simulink model "Experiment_cs"  (Simulink 8.4)
settings: Solver=ode5  SolverMode=SingleTasking  StartTime=0.0  StopTime=inf  FixedStep=1/100  RelTol=1e-3
PreLoadFcn:
  | mbxruntime.callbacks.PreLoadFcn(bdroot);
PostLoadFcn:
  | mbxruntime.callbacks.PostLoadFcn(bdroot);
InitFcn:
  | mbxruntime.callbacks.InitFcn(bdroot);
StartFcn:
  | mbxruntime.callbacks.StartFcn(bdroot);
StopFcn:
  | mbxruntime.callbacks.StopFcn(bdroot);
undefined symbols (not defined in the file or in its folder): dfreq, gray, InitImageOutputDir, Rec, SDTV, strel
libraries: simulink x79, visiontextngfix x30, simulink_extras x23, PreScanSimulinkLibrary x20, visionconversions x6, visionsinks x4, PreScanUsefulBlocks x3, visionstatistics x2, visionmorphops x2, visionanalysis x2, simulink_need_slupdate x2
(part 10 of 11)

== system Experiment_cs/Audi_A8_1/ENABLED/Dynamics_Simple/Chassis/Bicycle_model_[XYZ]/X_Motion/BrakeSystem ==
  vx_[ms-1] : Inport
  BrakePressure_[bar] : Inport  Port=2
  Gain : Gain  Gain=1/p.Rw
  Saturation : Saturate  UpperLimit=p.PBrakeMax  LowerLimit=0
  Saturation1 : Saturate  UpperLimit=5/15  LowerLimit=-5/15
  Sign : Signum
  "[ms-1] 2 [rads-1]" : Gain  Gain=1/p.Rw  SaturateOnIntegerOverflow=on  OutDataTypeStr=Inherit: Same as input  ParamDataTypeStr=Inherit: Same as input
  braking Q factor : Gain  Gain=p.Qfac  SaturateOnIntegerOverflow=on  OutDataTypeStr=Inherit: Same as input  ParamDataTypeStr=Inherit: Same as input
  signed load1 : Product  SaturateOnIntegerOverflow=on  InputSameDT=on  OutDataTypeStr=Inherit: Same as first input
  BrakeForce : Outport
  BrakeTorqueAbs : Outport  Port=2
  wires:
  braking Q factor/1 -> BrakeTorqueAbs/1, Gain/1
  BrakePressure_[bar]/1 -> Saturation/1
  Saturation/1 -> braking Q factor/1
  vx_[ms-1]/1 -> "[ms-1] 2 [rads-1]"/1
  Saturation1/1 -> Sign/1
  "[ms-1] 2 [rads-1]"/1 -> Saturation1/1
  Sign/1 -> signed load1/2  "sign"
  signed load1/1 -> BrakeForce/1
  Gain/1 -> signed load1/1

== system Experiment_cs/Audi_A8_1/ENABLED/Dynamics_Simple/Chassis/Bicycle_model_[XYZ]/X_Motion/Configurable Subsystem ==
  In1 : Inport
  In2 : Inport  Port=2
  In3 : Inport  Port=3
  Integrator : Integrator  ExternalReset=level  InitialConditionSource=external
  Out1 : Outport
  wires:
  In1/1 -> Integrator/1
  In2/1 -> Integrator/2
  In3/1 -> Integrator/3
  Integrator/1 -> Out1/1

== system Experiment_cs/Audi_A8_1/ENABLED/Dynamics_Simple/Chassis/Bicycle_model_[XYZ]/X_Motion/Configurable Subsystem1 ==
  In1 : Inport
  Torsional damping : TransferFcn  Denominator=[0.1 1]
  Out1 : Outport
  wires:
  In1/1 -> Torsional damping/1
  Torsional damping/1 -> Out1/1

== system Experiment_cs/Audi_A8_1/ENABLED/Dynamics_Simple/Chassis/Bicycle_model_[XYZ]/X_Motion/Max RPM and zero- velocity detection ==
  note: Set to zero after infinite small time-step
  note: Zero velocity detection
  ax : Inport
  Drive Torque : Inport  Port=2
  Brake Torque : Inport  Port=3
  v0 : Inport  Port=4
  vx : Inport  Port=5
  Abs : Abs
  Abs1 : Abs
  Compare To Zero : simulink/Logic and Bit Operations/Compare To Zero  relop=<=  OutDataTypeStr=boolean  ZeroCross=off
  Compare To Zero1 : simulink/Logic and Bit Operations/Compare To Zero  relop=>=  OutDataTypeStr=boolean  ZeroCross=off
  Compare To Zero2 : simulink/Logic and Bit Operations/Compare To Zero  relop=>=  OutDataTypeStr=boolean  ZeroCross=off
  Compare To Zero3 : simulink/Logic and Bit Operations/Compare To Zero  relop=<=  OutDataTypeStr=boolean  ZeroCross=off
  Configurable Subsystem : Subsystem  BlockChoice=Step  mask{ComputationMode=ComputationMode}
      mask prompts: ComputationMode "Compuation mode:"
      mask init:
      | SetComputationMode(gcb,ComputationMode);
      settings: AttributesFormatString=%<BlockChoice>  OpenFcn=BringToFront(gcb);  MemberBlocks=Discrete Step,Step
      settings: TemplateBlock=|
      | PreScanSimulinkLibrary/Configurable Subsystems/Step Function/Configurable
      | Subsystem
  Constant : Constant
  Constant1 : Constant
  Logical Operator : Logic  AllPortsSameDT=off  OutDataTypeStr=boolean
  Logical Operator1 : Logic  AllPortsSameDT=off  OutDataTypeStr=boolean
  Logical Operator2 : Logic  Operator=NOT  AllPortsSameDT=off  OutDataTypeStr=boolean
  Logical Operator3 : Logic  AllPortsSameDT=off  OutDataTypeStr=boolean
  Logical Operator4 : Logic  Operator=OR  AllPortsSameDT=off  OutDataTypeStr=boolean
  Memory : Memory
  Memory1 : Memory
  Memory2 : Memory
  Product : Product  RndMeth=Zero
  Relational Operator : RelationalOperator  Operator=<  OutDataTypeStr=boolean
  SR-Memory : Subsystem
  Sum : Sum  Inputs=|-+
  Switch : Switch  Criteria=u2 ~= 0  Threshold=0.5
  ax is 0 : Constant  Value=0
  ax_out : Outport
  vx_reset : Outport  Port=2
  x0 : Outport  Port=3
  wires:
  Logical Operator4/1 -> Logical Operator1/1
  vx/1 -> Compare To Zero/1, Compare To Zero2/1, Memory2/1, Memory/1  "vx"
  Memory2/1 -> Compare To Zero3/1
  Compare To Zero2/1 -> Logical Operator3/1
  Compare To Zero3/1 -> Logical Operator3/2
  Logical Operator3/1 -> Logical Operator4/2  "zero-crossing backward"
  Memory/1 -> Compare To Zero1/1
  Compare To Zero/1 -> Logical Operator/1
  Compare To Zero1/1 -> Logical Operator/2
  Logical Operator/1 -> Logical Operator4/1  "zero-crossing forward"
  Abs/1 -> Relational Operator/1
  Abs1/1 -> Relational Operator/2
  Drive Torque/1 -> Abs/1
  Brake Torque/1 -> Abs1/1
  Relational Operator/1 -> Logical Operator1/2, Logical Operator2/1
  Logical Operator1/1 -> SR-Memory/2(Set)
  Constant/1 -> SR-Memory/1(Signal)
  Logical Operator2/1 -> SR-Memory/3(Reset)
  SR-Memory/1(Out) -> Sum/1, Memory1/1
  Switch/1 -> ax_out/1
  Sum/1 -> Switch/2
  ax is 0/1 -> Switch/3
  Constant1/1 -> Sum/2
  v0/1 -> Product/1
  Product/1 -> x0/1
  Configurable Subsystem/1(Out1) -> Product/2
  ax/1 -> Switch/1  "ax"
  Memory1/1 -> vx_reset/1  "vx"

== system Experiment_cs/Audi_A8_1/ENABLED/Dynamics_Simple/Chassis/Bicycle_model_[XYZ]/Y & Yaw_Motion/Configurable Subsystem ==
  In1 : Inport
  In2 : Inport  Port=2
  Integrator : Integrator  ExternalReset=level
  Out1 : Outport
  wires:
  In1/1 -> Integrator/1
  In2/1 -> Integrator/2
  Integrator/1 -> Out1/1

== system Experiment_cs/Audi_A8_1/ENABLED/Dynamics_Simple/Chassis/Bicycle_model_[XYZ]/Y & Yaw_Motion/Configurable Subsystem1 ==
  In1 : Inport
  Integrator : Integrator
  Out1 : Outport
  wires:
  In1/1 -> Integrator/1
  Integrator/1 -> Out1/1

== system Experiment_cs/Audi_A8_1/ENABLED/Dynamics_Simple/Chassis/Bicycle_model_[XYZ]/Y & Yaw_Motion/Configurable Subsystem2 ==
  In1 : Inport
  In2 : Inport  Port=2
  Integrator : Integrator  ExternalReset=level
  Out1 : Outport
  wires:
  In1/1 -> Integrator/1
  In2/1 -> Integrator/2
  Integrator/1 -> Out1/1

== system Experiment_cs/Audi_A8_1/ENABLED/Dynamics_Simple/Chassis/Bicycle_model_[XYZ]/Z, Pitch_Motion & Roll_Motion/Configurable Subsystem ==
  In1 : Inport
  Integrator : Integrator  LimitOutput=on  UpperSaturationLimit=5*pi/180  LowerSaturationLimit=-5*pi/180
  Out1 : Outport
  wires:
  In1/1 -> Integrator/1
  Integrator/1 -> Out1/1

== system Experiment_cs/Audi_A8_1/ENABLED/Dynamics_Simple/Chassis/Bicycle_model_[XYZ]/Z, Pitch_Motion & Roll_Motion/Configurable Subsystem1 ==
  In1 : Inport
  Integrator : Integrator
  Out1 : Outport
  wires:
  In1/1 -> Integrator/1
  Integrator/1 -> Out1/1

== system Experiment_cs/Audi_A8_1/ENABLED/Dynamics_Simple/Chassis/Bicycle_model_[XYZ]/Z, Pitch_Motion & Roll_Motion/Configurable Subsystem2 ==
  In1 : Inport
  Integrator : Integrator
  Out1 : Outport
  wires:
  In1/1 -> Integrator/1
  Integrator/1 -> Out1/1

== system Experiment_cs/Audi_A8_1/ENABLED/Dynamics_Simple/Chassis/Bicycle_model_[XYZ]/Z, Pitch_Motion & Roll_Motion/Configurable Subsystem3 ==
  In1 : Inport
  Integrator : Integrator
  Out1 : Outport
  wires:
  In1/1 -> Integrator/1
  Integrator/1 -> Out1/1

== system Experiment_cs/Audi_A8_1/ENABLED/Dynamics_Simple/Chassis/Bicycle_model_[XYZ]/Z, Pitch_Motion & Roll_Motion/Configurable Subsystem4 ==
  In1 : Inport
  Integrator : Integrator
  Out1 : Outport
  wires:
  In1/1 -> Integrator/1
  Integrator/1 -> Out1/1

== system Experiment_cs/Audi_A8_1/ENABLED/Dynamics_Simple/Chassis/Bicycle_model_[XYZ]/Z, Pitch_Motion & Roll_Motion/Configurable Subsystem5 ==
  In1 : Inport
  Integrator : Integrator
  Out1 : Outport
  wires:
  In1/1 -> Integrator/1
  Integrator/1 -> Out1/1

== system Experiment_cs/Audi_A8_1/ENABLED/Dynamics_Simple/Chassis/Bicycle_model_[XYZ]/Z, Pitch_Motion & Roll_Motion/Configurable Subsystem9 ==
  In1 : Inport
  Derivative : Derivative
  Out1 : Outport
  wires:
  In1/1 -> Derivative/1
  Derivative/1 -> Out1/1

== system Experiment_cs/Audi_A8_1/ENABLED/Dynamics_Simple/Chassis/FrontTyre/AlphaFront/Enabled Subsystem ==
  In : Inport
  Enable : EnablePort  PropagateVarSize=During execution
  AlphaFront : Fcn  Expr=-atan( (u(2)+u(3)*p.a)/u(1) )
  Alpha : Outport  OutputWhenDisabled=reset  InitialOutput=[0]
  wires:
  AlphaFront/1 -> Alpha/1
  In/1 -> AlphaFront/1

== system Experiment_cs/Audi_A8_1/ENABLED/Dynamics_Simple/Chassis/RearTyre/AlphaRear/Enabled Subsystem ==
  In : Inport
  Enable : EnablePort  PropagateVarSize=During execution
  AlphaRear : Fcn  Expr=-atan( (u(2)-u(3)*p.b)/u(1) )
  Alpha : Outport  OutputWhenDisabled=reset  InitialOutput=[0]
  wires:
  AlphaRear/1 -> Alpha/1
  In/1 -> AlphaRear/1

== system Experiment_cs/Audi_A8_1/ENABLED/Trajectories/Traj2State1/Traj2State2/Traj2MuxState_Ext/demux ==
  traj : Inport
  Demux : Demux  Outputs=18
  x : Outport
  y : Outport  Port=2
  z : Outport  Port=3
  velx : Outport  Port=4
  vely : Outport  Port=5
  velz : Outport  Port=6
  R : Outport  Port=7
  P : Outport  Port=8
  Y : Outport  Port=9
  velR : Outport  Port=10
  velP : Outport  Port=11
  velY : Outport  Port=12
  accx : Outport  Port=13
  accy : Outport  Port=14
  accz : Outport  Port=15
  accR : Outport  Port=16
  accP : Outport  Port=17
  accY : Outport  Port=18
  wires:
  Demux/18 -> accY/1
  Demux/17 -> accP/1
  Demux/16 -> accR/1
  Demux/15 -> accz/1
  Demux/14 -> accy/1
  Demux/13 -> accx/1
  Demux/12 -> velY/1
  Demux/11 -> velP/1
  Demux/10 -> velR/1
  Demux/9 -> velz/1
  Demux/8 -> vely/1
  Demux/7 -> velx/1
  Demux/6 -> Y/1
  Demux/5 -> P/1
  traj/1 -> Demux/1
  Demux/4 -> R/1
  Demux/3 -> z/1
  Demux/2 -> y/1
  Demux/1 -> x/1

== system Experiment_cs/BMW_Z3_1/ENABLED/Dynamics_Simple/Chassis/Bicycle_model_[XYZ]/X_Motion/Air&RoadResistance ==
  vx_[ms-1] : Inport
  Gain : Gain  Gain=1/p.Rw
  Road & Aerodyn Resistances : Fcn  Expr=p.Rroad + p.Rair*u^2
  Saturation1 : Saturate  UpperLimit=5/15  LowerLimit=-5/15
  Sign : Signum
  "[ms-1] 2 [rads-1]" : Gain  Gain=1/p.Rw  SaturateOnIntegerOverflow=on  OutDataTypeStr=Inherit: Same as input  ParamDataTypeStr=Inherit: Same as input
  signed load1 : Product  SaturateOnIntegerOverflow=on  InputSameDT=on  OutDataTypeStr=Inherit: Same as first input
  Resistance_Force : Outport
  wires:
  signed load1/1 -> Resistance_Force/1  "F_[N]"
  vx_[ms-1]/1 -> Road & Aerodyn Resistances/1, "[ms-1] 2 [rads-1]"/1
  Saturation1/1 -> Sign/1
  "[ms-1] 2 [rads-1]"/1 -> Saturation1/1
  Road & Aerodyn Resistances/1 -> Gain/1  "ResistanceTorque_[Nm]"
  Sign/1 -> signed load1/2  "sign"
  Gain/1 -> signed load1/1  "Resistance Force_[N]"

== system Experiment_cs/BMW_Z3_1/ENABLED/Dynamics_Simple/Chassis/Bicycle_model_[XYZ]/X_Motion/BrakeSystem ==
  vx_[ms-1] : Inport
  BrakePressure_[bar] : Inport  Port=2
  Gain : Gain  Gain=1/p.Rw
  Saturation : Saturate  UpperLimit=p.PBrakeMax  LowerLimit=0
  Saturation1 : Saturate  UpperLimit=5/15  LowerLimit=-5/15
  Sign : Signum
  "[ms-1] 2 [rads-1]" : Gain  Gain=1/p.Rw  SaturateOnIntegerOverflow=on  OutDataTypeStr=Inherit: Same as input  ParamDataTypeStr=Inherit: Same as input
  braking Q factor : Gain  Gain=p.Qfac  SaturateOnIntegerOverflow=on  OutDataTypeStr=Inherit: Same as input  ParamDataTypeStr=Inherit: Same as input
  signed load1 : Product  SaturateOnIntegerOverflow=on  InputSameDT=on  OutDataTypeStr=Inherit: Same as first input
  BrakeForce : Outport
  BrakeTorqueAbs : Outport  Port=2
  wires:
  braking Q factor/1 -> BrakeTorqueAbs/1, Gain/1
  BrakePressure_[bar]/1 -> Saturation/1
  Saturation/1 -> braking Q factor/1
  vx_[ms-1]/1 -> "[ms-1] 2 [rads-1]"/1
  Saturation1/1 -> Sign/1
  "[ms-1] 2 [rads-1]"/1 -> Saturation1/1
  Sign/1 -> signed load1/2  "sign"
  signed load1/1 -> BrakeForce/1
  Gain/1 -> signed load1/1

== system Experiment_cs/BMW_Z3_1/ENABLED/Dynamics_Simple/Chassis/Bicycle_model_[XYZ]/X_Motion/Configurable Subsystem ==
  In1 : Inport
  In2 : Inport  Port=2
  In3 : Inport  Port=3
  Integrator : Integrator  ExternalReset=level  InitialConditionSource=external
  Out1 : Outport
  wires:
  In1/1 -> Integrator/1
  In2/1 -> Integrator/2
  In3/1 -> Integrator/3
  Integrator/1 -> Out1/1

== system Experiment_cs/BMW_Z3_1/ENABLED/Dynamics_Simple/Chassis/Bicycle_model_[XYZ]/X_Motion/Configurable Subsystem1 ==
  In1 : Inport
  Torsional damping : TransferFcn  Denominator=[0.1 1]
  Out1 : Outport
  wires:
  In1/1 -> Torsional damping/1
  Torsional damping/1 -> Out1/1

== system Experiment_cs/BMW_Z3_1/ENABLED/Dynamics_Simple/Chassis/Bicycle_model_[XYZ]/X_Motion/Max RPM and zero- velocity detection ==
  note: Set to zero after infinite small time-step
  note: Zero velocity detection
  ax : Inport
  Drive Torque : Inport  Port=2
  Brake Torque : Inport  Port=3
  v0 : Inport  Port=4
  vx : Inport  Port=5
  Abs : Abs
  Abs1 : Abs
  Compare To Zero : simulink/Logic and Bit Operations/Compare To Zero  relop=<=  OutDataTypeStr=boolean  ZeroCross=off
  Compare To Zero1 : simulink/Logic and Bit Operations/Compare To Zero  relop=>=  OutDataTypeStr=boolean  ZeroCross=off
  Compare To Zero2 : simulink/Logic and Bit Operations/Compare To Zero  relop=>=  OutDataTypeStr=boolean  ZeroCross=off
  Compare To Zero3 : simulink/Logic and Bit Operations/Compare To Zero  relop=<=  OutDataTypeStr=boolean  ZeroCross=off
  Configurable Subsystem : Subsystem  BlockChoice=Step  mask{ComputationMode=ComputationMode}
      mask prompts: ComputationMode "Compuation mode:"
      mask init:
      | SetComputationMode(gcb,ComputationMode);
      settings: AttributesFormatString=%<BlockChoice>  OpenFcn=BringToFront(gcb);  MemberBlocks=Discrete Step,Step
      settings: TemplateBlock=|
      | PreScanSimulinkLibrary/Configurable Subsystems/Step Function/Configurable
      | Subsystem
  Constant : Constant
  Constant1 : Constant
  Logical Operator : Logic  AllPortsSameDT=off  OutDataTypeStr=boolean
  Logical Operator1 : Logic  AllPortsSameDT=off  OutDataTypeStr=boolean
  Logical Operator2 : Logic  Operator=NOT  AllPortsSameDT=off  OutDataTypeStr=boolean
  Logical Operator3 : Logic  AllPortsSameDT=off  OutDataTypeStr=boolean
  Logical Operator4 : Logic  Operator=OR  AllPortsSameDT=off  OutDataTypeStr=boolean
  Memory : Memory
  Memory1 : Memory
  Memory2 : Memory
  Product : Product  RndMeth=Zero
  Relational Operator : RelationalOperator  Operator=<  OutDataTypeStr=boolean
  SR-Memory : Subsystem
  Sum : Sum  Inputs=|-+
  Switch : Switch  Criteria=u2 ~= 0  Threshold=0.5
  ax is 0 : Constant  Value=0
  ax_out : Outport
  vx_reset : Outport  Port=2
  x0 : Outport  Port=3
  wires:
  Logical Operator4/1 -> Logical Operator1/1
  vx/1 -> Compare To Zero/1, Compare To Zero2/1, Memory2/1, Memory/1  "vx"
  Memory2/1 -> Compare To Zero3/1
  Compare To Zero2/1 -> Logical Operator3/1
  Compare To Zero3/1 -> Logical Operator3/2
  Logical Operator3/1 -> Logical Operator4/2  "zero-crossing backward"
  Memory/1 -> Compare To Zero1/1
  Compare To Zero/1 -> Logical Operator/1
  Compare To Zero1/1 -> Logical Operator/2
  Logical Operator/1 -> Logical Operator4/1  "zero-crossing forward"
  Abs/1 -> Relational Operator/1
  Abs1/1 -> Relational Operator/2
  Drive Torque/1 -> Abs/1
  Brake Torque/1 -> Abs1/1
  Relational Operator/1 -> Logical Operator1/2, Logical Operator2/1
  Logical Operator1/1 -> SR-Memory/2(Set)
  Constant/1 -> SR-Memory/1(Signal)
  Logical Operator2/1 -> SR-Memory/3(Reset)
  SR-Memory/1(Out) -> Sum/1, Memory1/1
  Switch/1 -> ax_out/1
  Sum/1 -> Switch/2
  ax is 0/1 -> Switch/3
  Constant1/1 -> Sum/2
  v0/1 -> Product/1
  Product/1 -> x0/1
  Configurable Subsystem/1(Out1) -> Product/2
  ax/1 -> Switch/1  "ax"
  Memory1/1 -> vx_reset/1  "vx"

== system Experiment_cs/BMW_Z3_1/ENABLED/Dynamics_Simple/Chassis/Bicycle_model_[XYZ]/Y & Yaw_Motion/Configurable Subsystem ==
  In1 : Inport
  In2 : Inport  Port=2
  Integrator : Integrator  ExternalReset=level
  Out1 : Outport
  wires:
  In1/1 -> Integrator/1
  In2/1 -> Integrator/2
  Integrator/1 -> Out1/1

== system Experiment_cs/BMW_Z3_1/ENABLED/Dynamics_Simple/Chassis/Bicycle_model_[XYZ]/Y & Yaw_Motion/Configurable Subsystem1 ==
  In1 : Inport
  Integrator : Integrator
  Out1 : Outport
  wires:
  In1/1 -> Integrator/1
  Integrator/1 -> Out1/1

== system Experiment_cs/BMW_Z3_1/ENABLED/Dynamics_Simple/Chassis/Bicycle_model_[XYZ]/Y & Yaw_Motion/Configurable Subsystem2 ==
  In1 : Inport
  In2 : Inport  Port=2
  Integrator : Integrator  ExternalReset=level
  Out1 : Outport
  wires:
  In1/1 -> Integrator/1
  In2/1 -> Integrator/2
  Integrator/1 -> Out1/1

== system Experiment_cs/BMW_Z3_1/ENABLED/Dynamics_Simple/Chassis/Bicycle_model_[XYZ]/Z, Pitch_Motion & Roll_Motion/Configurable Subsystem ==
  In1 : Inport
  Integrator : Integrator  LimitOutput=on  UpperSaturationLimit=5*pi/180  LowerSaturationLimit=-5*pi/180
  Out1 : Outport
  wires:
  In1/1 -> Integrator/1
  Integrator/1 -> Out1/1

== system Experiment_cs/BMW_Z3_1/ENABLED/Dynamics_Simple/Chassis/Bicycle_model_[XYZ]/Z, Pitch_Motion & Roll_Motion/Configurable Subsystem1 ==
  In1 : Inport
  Integrator : Integrator
  Out1 : Outport
  wires:
  In1/1 -> Integrator/1
  Integrator/1 -> Out1/1

== system Experiment_cs/BMW_Z3_1/ENABLED/Dynamics_Simple/Chassis/Bicycle_model_[XYZ]/Z, Pitch_Motion & Roll_Motion/Configurable Subsystem2 ==
  In1 : Inport
  Integrator : Integrator
  Out1 : Outport
  wires:
  In1/1 -> Integrator/1
  Integrator/1 -> Out1/1

== system Experiment_cs/BMW_Z3_1/ENABLED/Dynamics_Simple/Chassis/Bicycle_model_[XYZ]/Z, Pitch_Motion & Roll_Motion/Configurable Subsystem3 ==
  In1 : Inport
  Integrator : Integrator
  Out1 : Outport
  wires:
  In1/1 -> Integrator/1
  Integrator/1 -> Out1/1

== system Experiment_cs/BMW_Z3_1/ENABLED/Dynamics_Simple/Chassis/Bicycle_model_[XYZ]/Z, Pitch_Motion & Roll_Motion/Configurable Subsystem4 ==
  In1 : Inport
  Integrator : Integrator
  Out1 : Outport
  wires:
  In1/1 -> Integrator/1
  Integrator/1 -> Out1/1

== system Experiment_cs/BMW_Z3_1/ENABLED/Dynamics_Simple/Chassis/Bicycle_model_[XYZ]/Z, Pitch_Motion & Roll_Motion/Configurable Subsystem5 ==
  In1 : Inport
  Integrator : Integrator
  Out1 : Outport
  wires:
  In1/1 -> Integrator/1
  Integrator/1 -> Out1/1

== system Experiment_cs/BMW_Z3_1/ENABLED/Dynamics_Simple/Chassis/Bicycle_model_[XYZ]/Z, Pitch_Motion & Roll_Motion/Configurable Subsystem9 ==
  In1 : Inport
  Derivative : Derivative
  Out1 : Outport
  wires:
  In1/1 -> Derivative/1
  Derivative/1 -> Out1/1

== system Experiment_cs/BMW_Z3_1/ENABLED/Dynamics_Simple/Chassis/FrontTyre/AlphaFront/Enabled Subsystem ==
  In : Inport
  Enable : EnablePort  PropagateVarSize=During execution
  AlphaFront : Fcn  Expr=-atan( (u(2)+u(3)*p.a)/u(1) )
  Alpha : Outport  OutputWhenDisabled=reset  InitialOutput=[0]
  wires:
  AlphaFront/1 -> Alpha/1
  In/1 -> AlphaFront/1

== system Experiment_cs/BMW_Z3_1/ENABLED/Dynamics_Simple/Chassis/RearTyre/AlphaRear/Enabled Subsystem ==
  In : Inport
  Enable : EnablePort  PropagateVarSize=During execution
  AlphaRear : Fcn  Expr=-atan( (u(2)-u(3)*p.b)/u(1) )
  Alpha : Outport  OutputWhenDisabled=reset  InitialOutput=[0]
  wires:
  AlphaRear/1 -> Alpha/1
  In/1 -> AlphaRear/1

== system Experiment_cs/BMW_Z3_1/ENABLED/Trajectories/Traj2State1/Traj2State2/Traj2MuxState_Ext/demux ==
  traj : Inport
  Demux : Demux  Outputs=18
  x : Outport
  y : Outport  Port=2
  z : Outport  Port=3
  velx : Outport  Port=4
  vely : Outport  Port=5
  velz : Outport  Port=6
  R : Outport  Port=7
  P : Outport  Port=8
  Y : Outport  Port=9
  velR : Outport  Port=10
  velP : Outport  Port=11
  velY : Outport  Port=12
  accx : Outport  Port=13
  accy : Outport  Port=14
  accz : Outport  Port=15
  accR : Outport  Port=16
  accP : Outport  Port=17
  accY : Outport  Port=18
  wires:
  Demux/18 -> accY/1
  Demux/17 -> accP/1
  Demux/16 -> accR/1
  Demux/15 -> accz/1
  Demux/14 -> accy/1
  Demux/13 -> accx/1
  Demux/12 -> velY/1
  Demux/11 -> velP/1
  Demux/10 -> velR/1
  Demux/9 -> velz/1
  Demux/8 -> vely/1
  Demux/7 -> velx/1
  Demux/6 -> Y/1
  Demux/5 -> P/1
  traj/1 -> Demux/1
  Demux/4 -> R/1
  Demux/3 -> z/1
  Demux/2 -> y/1
  Demux/1 -> x/1

== system Experiment_cs/Man_200_1/ENABLED/Trajectories/Traj2State1/Traj2State2/Traj2MuxState_Ext/demux ==
  traj : Inport
  Demux : Demux  Outputs=18
  x : Outport
  y : Outport  Port=2
  z : Outport  Port=3
  velx : Outport  Port=4
  vely : Outport  Port=5
  velz : Outport  Port=6
  R : Outport  Port=7
  P : Outport  Port=8
  Y : Outport  Port=9
  velR : Outport  Port=10
  velP : Outport  Port=11
  velY : Outport  Port=12
  accx : Outport  Port=13
  accy : Outport  Port=14
  accz : Outport  Port=15
  accR : Outport  Port=16
  accP : Outport  Port=17
  accY : Outport  Port=18
  wires:
  Demux/18 -> accY/1
  Demux/17 -> accP/1
  Demux/16 -> accR/1
  Demux/15 -> accz/1
  Demux/14 -> accy/1
  Demux/13 -> accx/1
  Demux/12 -> velY/1
  Demux/11 -> velP/1
  Demux/10 -> velR/1
  Demux/9 -> velz/1
  Demux/8 -> vely/1
  Demux/7 -> velx/1
  Demux/6 -> Y/1
  Demux/5 -> P/1
  traj/1 -> Demux/1
  Demux/4 -> R/1
  Demux/3 -> z/1
  Demux/2 -> y/1
  Demux/1 -> x/1

== system Experiment_cs/Audi_A8_1/ENABLED/Dynamics_Simple/Chassis/Bicycle_model_[XYZ]/X_Motion/Max RPM and zero- velocity detection/Configurable Subsystem ==
  Step : Step  Time=0.0001  Before=1  After=0  SampleTime=0
  Out1 : Outport
  wires:
  Step/1 -> Out1/1

== system Experiment_cs/Audi_A8_1/ENABLED/Dynamics_Simple/Chassis/Bicycle_model_[XYZ]/X_Motion/Max RPM and zero- velocity detection/SR-Memory ==
  Signal : Inport
  Set : Inport  Port=2
  Reset : Inport  Port=3
  Constant : Constant  Value=0
  Detect Rise Positive : simulink/Logic and Bit Operations/Detect Rise Positive  vinit=0  InputProcessing=Inherited  OutDataTypeStr=uint8
  Detect Rise Positive1 : simulink/Logic and Bit Operations/Detect Rise Positive  vinit=0  InputProcessing=Inherited  OutDataTypeStr=uint8
  Manual Switch : ManualSwitch
  Manual Switch1 : ManualSwitch
  Switch : Switch  Criteria=u2 ~= 0
  Switch1 : Switch  Criteria=u2 ~= 0
  Unit Delay : UnitDelay  SampleTime=-1
  Out : Outport
  wires:
  Constant/1 -> Switch1/1
  Switch/1 -> Switch1/3
  Switch1/1 -> Unit Delay/1, Out/1
  Manual Switch1/1 -> Switch1/2
  Reset/1 -> Manual Switch1/2, Detect Rise Positive1/1
  Detect Rise Positive1/1 -> Manual Switch1/1
  Signal/1 -> Switch/1
  Unit Delay/1 -> Switch/3
  Set/1 -> Detect Rise Positive/1, Manual Switch/2
  Detect Rise Positive/1 -> Manual Switch/1
  Manual Switch/1 -> Switch/2

== system Experiment_cs/BMW_Z3_1/ENABLED/Dynamics_Simple/Chassis/Bicycle_model_[XYZ]/X_Motion/Max RPM and zero- velocity detection/Configurable Subsystem ==
  Step : Step  Time=0.0001  Before=1  After=0  SampleTime=0
  Out1 : Outport
  wires:
  Step/1 -> Out1/1

== system Experiment_cs/BMW_Z3_1/ENABLED/Dynamics_Simple/Chassis/Bicycle_model_[XYZ]/X_Motion/Max RPM and zero- velocity detection/SR-Memory ==
  Signal : Inport
  Set : Inport  Port=2
  Reset : Inport  Port=3
  Constant : Constant  Value=0
  Detect Rise Positive : simulink/Logic and Bit Operations/Detect Rise Positive  vinit=0  InputProcessing=Inherited  OutDataTypeStr=uint8
  Detect Rise Positive1 : simulink/Logic and Bit Operations/Detect Rise Positive  vinit=0  InputProcessing=Inherited  OutDataTypeStr=uint8
  Manual Switch : ManualSwitch
  Manual Switch1 : ManualSwitch
  Switch : Switch  Criteria=u2 ~= 0
  Switch1 : Switch  Criteria=u2 ~= 0
  Unit Delay : UnitDelay  SampleTime=-1
  Out : Outport
  wires:
  Constant/1 -> Switch1/1
  Switch/1 -> Switch1/3
  Switch1/1 -> Unit Delay/1, Out/1
  Manual Switch1/1 -> Switch1/2
  Reset/1 -> Manual Switch1/2, Detect Rise Positive1/1
  Detect Rise Positive1/1 -> Manual Switch1/1
  Signal/1 -> Switch/1
  Unit Delay/1 -> Switch/3
  Set/1 -> Detect Rise Positive/1, Manual Switch/2
  Detect Rise Positive/1 -> Manual Switch/1
  Manual Switch/1 -> Switch/2

== matlab function BMW_Z3_1/ENABLED/PathFollower_1/CTRL REFERENCES/Find Reference Point (pref) on Trajectory closest to PVP Point (pvp)/eml_find_closest_trajectory_points ==
  data: pref output double; Actor_traj_distance output double; Actor_traj_angle output double; pvp input double; TrajOffset_x_y_Y input double size=3; ActorOffset_Left_Right input double; p0 input double size=3; Traj_x parameter double; Traj_y parameter double
function [pref,Actor_traj_distance,Actor_traj_angle]  = eml_find_closest_trajectory_points(pvp,TrajOffset_x_y_Y,ActorOffset_Left_Right,p0,Traj_x,Traj_y)

[pref,Actor_traj_distance,Actor_traj_angle] = emlfcn_find_closest_trajectory_points(pvp,TrajOffset_x_y_Y,ActorOffset_Left_Right,p0,Traj_x,Traj_y,1);

end % end function

== matlab function BMW_Z3_1/ENABLED/PathFollower_1/DELTA CTRL/Calculate preview angle/eml_preview_angle_and_distance ==
  data: pvp input double; alpha output double; pref input double; p0 input double
function alpha = eml_preview_angle_and_distance(pvp, pref, p0)
%#eml

alpha = emlfcn_preview_angle_and_distance(pvp, pref, p0);

% end function

== matlab function Audi_A8_1/ENABLED/PPS Model/Pedestrian detection/Blob Analysis/PEDES2 ==
  data: inpoints output double; pts input double
function inpoints= points(pts)
%#eml
inpoints = pts;
inpoints(1, :)=pts(2, :);
inpoints(2, :)=pts(1, :);
inpoints(3, :)=pts(4, :);
inpoints(4, :)=pts(3, :);

for i = 1 : size(inpoints, 2)
    if inpoints(1, i) ~= -1
        inpoints(1, i)=inpoints(1, i) -1;
    end
    if inpoints(2, i) ~= -1
        inpoints(2, i)=inpoints(2, i) -1;
    end
end

== matlab function Audi_A8_1/ENABLED/PPS Model/Pedestrian detection/PEDES3 ==
  data: inpoints output double; pts input double
function inpoints= points(pts)
%#eml
inpoints = pts;
inpoints(1, :)=pts(2, :);
inpoints(2, :)=pts(1, :);
inpoints(3, :)=pts(4, :);
inpoints(4, :)=pts(3, :);

for i = 1 : size(inpoints, 2)
    if inpoints(1, i) ~= -1
        inpoints(1, i)=inpoints(1, i) +1;
    end
    if inpoints(2, i) ~= -1
        inpoints(2, i)=inpoints(2, i) +1;
    end
end

== matlab function Audi_A8_1/ENABLED/PPS Model/Pedestrian detection/PEDES4 ==
  data: inpoints output double; pts input double
function inpoints= points(pts)
%#eml
inpoints = pts;
for i=1:size(pts,1)
    for j=1:2
         inpoints(i,j)=pts(i,j)+1;
    end
     for j=3:4
         inpoints(i,j)=pts(i,j)-1;
    end
end

== matlab function Audi_A8_1/ENABLED/PPS Model/Pedestrian detection/PEDES6 ==
  data: inpoints output double; pts input double
function inpoints= points(pts)
%#eml
inpoints = pts;
inpoints(1, :)=pts(2, :);
inpoints(2, :)=pts(1, :);

for i = 1 : size(inpoints, 2)
    if inpoints(1, i) ~= -1
        inpoints(1, i)=inpoints(1, i) +1;
    end
    if inpoints(2, i) ~= -1
        inpoints(2, i)=inpoints(2, i) +1;
    end
end

== matlab function Audi_A8_1/ENABLED/PPS Model/Pedestrian detection/Blob Analysis/PEDES1 ==
  data: inpoints output double; pts input double
function inpoints= points(pts)
%#eml
inpoints = pts;
inpoints(1, :)=pts(2, :);
inpoints(2, :)=pts(1, :);

for i = 1 : size(inpoints, 2)
    if inpoints(1, i) ~= -1
        inpoints(1, i)=inpoints(1, i) +1;
    end
    if inpoints(2, i) ~= -1
        inpoints(2, i)=inpoints(2, i) +1;
    end
end

== matlab function Audi_A8_1/ENABLED/PPS Model/Pedestrian detection/POSITION ==
  data: flag input double size=TISdet; theta input double size=TISdet; posit output double; range input double; xs_m output double; ys_m output double; TISdet parameter double; TISMaxRange parameter double
function [posit,xs_m,ys_m]= positt(flag,theta,range,TISdet, TISMaxRange)
%#codegen
xposit = zeros(1,TISdet);
yposit = zeros(1,TISdet);
posit = zeros(2,TISdet);
xs_m = zeros(1,TISdet);
ys_m = zeros(1,TISdet);
X_offset = 3.9 - 1.9;                                   %Offset Between Camera and Radar Positions
Z_offset = 0.42 - 1.28;                                 %Offset Between Camera and Radar Positions

f = 0.0075;                                             %Focal Length
sx = 0.0048;                                            %Pixel Width
%Maximum Camera Cooridnates%
u_max = TISMaxRange * sin(23.1*pi/180);                          %radar range = 40m, camera fov = 46.2 degrees 
v_max = TISMaxRange * cos(23.1*pi/180);

for i=1:TISdet
    if (flag(i)==0) || (theta(i)==0)
        xposit(i) = 0;
        posit(1,i) = 0;
    elseif (flag(i)~=0)
        theta_aux = -theta(i);      
        
        X = range(i)*cos(theta_aux*pi/180);
        Y = range(i)*sin(theta_aux*pi/180);
        
        xs_m(i) = Y;        
        ys_m(i) = X;
        %Camera 3-D Coordinates%
        X_c = X + X_offset;
        Y_c = Y;

        %Camera Pixel Coordinates%
        u_r_new = (Y*f*500)/(sx*u_max);
      
        %Conversion of xc to pixel value%
        xposit(i)= 250 + u_r_new;
        yposit(i)=188;
    end
     posit(2,i)=round(xposit(i));
     posit(1,i)=round(yposit(i));
end

== matlab function Audi_A8_1/ENABLED/PPS Model/Pedestrian detection/PEDES8 ==
  data: inpoints output double; pts input double
function inpoints= points(pts)
%#eml
inpoints = pts;
inpoints(1, :)=pts(2, :);
inpoints(2, :)=pts(1, :);

for i = 1 : size(inpoints, 2)
    if inpoints(1, i) ~= -1
        inpoints(1, i)=inpoints(1, i) +1;
    end
    if inpoints(2, i) ~= -1
        inpoints(2, i)=inpoints(2, i) +1;
    end
end

== matlab function Audi_A8_1/ENABLED/PPS Model/Pedestrian detection/PEDES9 ==
  data: inpoints output double; pts input double
function inpoints= points(pts)
%#eml
inpoints = pts;
for i=0:(size(pts,1)/2-1)    
    inpoints(2*i+1)=pts(2*i+2);
    inpoints(2*i+2)=pts(2*i+1);
end

== matlab function Audi_A8_1/ENABLED/PPS Model/Pedestrian detection/PEDES10 ==
  data: inpoints output double; pts input double
function inpoints= points(pts)
%#eml
inpoints = pts;
inpoints(1, :)=pts(2, :);
inpoints(2, :)=pts(1, :);

for i = 1 : size(inpoints, 2)
    if inpoints(1, i) ~= -1
        inpoints(1, i)=inpoints(1, i) +1;
    end
    if inpoints(2, i) ~= -1
        inpoints(2, i)=inpoints(2, i) +1;
    end
end

== matlab function Audi_A8_1/ENABLED/PPS Model/Pedestrian detection/Blob Analysis/PEDES4 ==
  data: inpoints output double; pts input double
function inpoints= points(pts)
%#eml
inpoints = pts;
inpoints(1, :)=pts(2, :);
inpoints(2, :)=pts(1, :);
inpoints(3, :)=pts(4, :);
inpoints(4, :)=pts(3, :);

for i = 1 : size(inpoints, 2)
    if inpoints(1, i) ~= -1
        inpoints(1, i)=inpoints(1, i) +1;
    end
    if inpoints(2, i) ~= -1
        inpoints(2, i)=inpoints(2, i) +1;
    end
end

== matlab function Audi_A8_1/ENABLED/PPS Model/Pedestrian detection/scaling_crop ==
  data: im input double; PosObj input double; X input double; Y input double; sub_im output double size=[375 500]; posObj_subim output double; im_x output double; im_y output double; liminf_x output double; liminf_y output double; rectangle output double
function [sub_im,posObj_subim,im_x,im_y,liminf_x, liminf_y,rectangle]=escaling(im,PosObj,X,Y)

minPx=size(im,2);
minPy=size(im,1);
maxPx=0;
maxPy=0;
detected=0;
mino=0;
maxo=0;
for i=1:size(PosObj,2)
    if PosObj(2,i)~=0
        if(PosObj(2,i)<minPx)
            minPx=PosObj(2,i);
            minPy=PosObj(1,i);
            mino=i;
        end
        if (PosObj(2,i)>maxPx)
            maxPx=PosObj(2,i);
            maxPy=PosObj(1,i);
            maxo=i;
        end
        detected=detected+1;
    end
end
if (detected==0)
    liminf_x=size(im,2);
    limsup_x=size(im,2);
    liminf_y=size(im,1);
    limsup_y=size(im,1);
 
 else
   
  %%For horizontal and vertical position
   
  if (mino~=0) 
    liminf_x= round(minPx-((40-round(1.6*Y(mino)))*2));
    liminf_y= round(minPy-((100-round(4.5*Y(mino)))*2));
    
  else
     liminf_x=1;
     liminf_y=1;
  end
   if (maxo~=0)   
    limsup_x= abs(round(maxPx+((40-round(1.6*Y(maxo)))*2)));
    limsup_y= abs(round(maxPy+((100-round(5*Y(maxo)))*2)));
   else
       limsup_x=size(im,2);
       limsup_y=size(im,1);
   end

end

  if (liminf_x<1)
         liminf_x=1;
  end
    
  if (limsup_x>size(im,2))
        limsup_x=size(im,2);
  end
    
  if (liminf_y<1)
       liminf_y=1;
  end
    
  if (limsup_y>=size(im,1))
       limsup_y=size(im,1);
  end
  
  if (liminf_y > size(im,1))
        liminf_y = size(im,1);
  end
    
   posObj_subim=zeros(2,size(PosObj,2));
   a=1;
    
    for i=1:size(PosObj,2)
        if (PosObj(2,i)~=0)
            posObj_subim(:,a)=[PosObj(1,i)-liminf_y;PosObj(2,i)-liminf_x];
            a=a+1;
        end
    end

sub_im=im(liminf_y:limsup_y,liminf_x:limsup_x);

if length( sub_im ) < 3
    sub_im = zeros(3,3,'uint8');
end


im_x=limsup_x-liminf_x;
im_y=limsup_y-liminf_y;
rectangle=[liminf_y liminf_x im_y im_x];

== matlab function Audi_A8_1/ENABLED/PPS Model/Pedestrian detection/Blob Analysis/MATLAB Function ==
  data: u input double; y output double
function y = fcn(u)
%#codegen

y = u(1:2, :);

== matlab function Audi_A8_1/ENABLED/PathFollower_1/CTRL REFERENCES/Find Reference Point (pref) on Trajectory closest to PVP Point (pvp)/eml_find_closest_trajectory_points ==
  data: pref output double; Actor_traj_distance output double; Actor_traj_angle output double; pvp input double; TrajOffset_x_y_Y input double size=3; ActorOffset_Left_Right input double; p0 input double size=3; Traj_x parameter double; Traj_y parameter double
function [pref,Actor_traj_distance,Actor_traj_angle]  = eml_find_closest_trajectory_points(pvp,TrajOffset_x_y_Y,ActorOffset_Left_Right,p0,Traj_x,Traj_y)

[pref,Actor_traj_distance,Actor_traj_angle] = emlfcn_find_closest_trajectory_points(pvp,TrajOffset_x_y_Y,ActorOffset_Left_Right,p0,Traj_x,Traj_y,1);

end % end function

== matlab function Audi_A8_1/ENABLED/PathFollower_1/DELTA CTRL/Calculate preview angle/eml_preview_angle_and_distance ==
  data: pvp input double; alpha output double; pref input double; p0 input double
function alpha = eml_preview_angle_and_distance(pvp, pref, p0)
%#eml

alpha = emlfcn_preview_angle_and_distance(pvp, pref, p0);

% end function

== matlab function Audi_A8_1/ENABLED/PPS Model/Pedestrian detection/Blob Analysis/PEDES3 ==
  data: inpoints output double; pts input double
function inpoints= points(pts)
%#eml
inpoints = pts;
inpoints(1, :)=pts(2, :);
inpoints(2, :)=pts(1, :);
for i = 1 : size(inpoints, 2)
    if inpoints(1, i) ~= -1
        inpoints(1, i)=inpoints(1, i) -1;
    end
    if inpoints(2, i) ~= -1
        inpoints(2, i)=inpoints(2, i) -1;
    end
end

== matlab function Audi_A8_1/ENABLED/PPS Model/Pedestrian detection/Blob Analysis/Embedded MATLAB Function1 ==
  data: centroid input double; centout output double; bbox input double; bboxout output double; majoraxis input double; minoraxis input double; orientation input double; eccentricity input double; label input double; label_out output double size=[400 550]; im_x input double; im_y input double; posObj_subim input double; liminf_x input double; liminf_y input double; posObj_im output double
function [centout,bboxout,label_out,posObj_im] = select_blobs(centroid,bbox,majoraxis,minoraxis,orientation,eccentricity,label,im_x,im_y,posObj_subim, liminf_x,liminf_y)
%#eml
a=1;
centroid=int32(centroid);
centout=int32(zeros(2,size(centroid,2)));
bboxout=int32(zeros(4,size(bbox,2)));
label_out=zeros(size(label,1),size(label,2));
posObj_im=posObj_subim;
for i=1:size(posObj_subim,2)
    posObj_im(:,i)=posObj_subim(:,i)+[liminf_y;liminf_x];
end

for i=1:size(orientation,2)
    touch=0;
    if orientation(1,i)>=180
         or_val=360-orientation(1,i);
     else
         or_val=orientation(1,i);
     end
     lr=bbox(1,i)+1;
     lh=lr+bbox(3,i)-1;
     lc=bbox(2,i)+1;
     lw=lc+bbox(4,i)-1;
      if (bbox(1,i)==0)
          touch=touch+1;
      end
      if (bbox(2,i)==0)
          touch=touch+1;
      end
      if(im_y-centroid(1,i)-(bbox(4,i)/2)<2)
          touch=touch+1;
      end
      if (im_x-centroid(2,i)-(bbox(3,i)/2)<2)
          touch=touch+1;
      end
     
     if (abs(or_val)>55)&&(abs(or_val)<145)&&((majoraxis(i)/minoraxis(i))>1.5)&&((majoraxis(i)/minoraxis(i))<3)&&(eccentricity(i)>0)&&(eccentricity(i)<1)&&(touch<2)
         bboxout(1:2,a)= bbox(1:2,i)+int32([liminf_y;liminf_x]);
         bboxout(3:4,a)= bbox(3:4,i);
         centout(:,a)= centroid(:,i)+int32([liminf_y;liminf_x]);
         label_out(lr:lh,lc:lw)=a;
         a=a+1;
     else
        label_out(lr:lh,lc:lw)=0;
     end
end

== matlab function Audi_A8_1/ENABLED/PPS Model/Pedestrian detection/PEDES7 ==
  data: inpoints output double; pts input double
function inpoints= points(pts)
%#eml
inpoints = pts;
inpoints(1, :)=pts(2, :);
inpoints(2, :)=pts(1, :);
inpoints(3, :)=pts(4, :);
inpoints(4, :)=pts(3, :);

for i = 1 : size(inpoints, 2)
    if inpoints(1, i) ~= -1
        inpoints(1, i)=inpoints(1, i) +1;
    end
    if inpoints(2, i) ~= -1
        inpoints(2, i)=inpoints(2, i) +1;
    end
end

== matlab function Audi_A8_1/ENABLED/PPS Model/Pedestrian detection/Blob Analysis/Embedded MATLAB Function2 ==
  data: nbboxout input double; label input double; r_label output double; color output double
function [r_label,color] = r_labels(nbboxout,label)
%#eml
n=size(nbboxout,2);
r_label=zeros(1,n);
color=zeros(1,n);
not_before=1;
a=1;
for i=1:size(label,1)
    for j=1:size(label,2)
        if (a==1)
            if (label(i,j)~=0)
                r_label(1,a)=label(i,j);
                a=a+1;
            end
        else
             if (label(i,j)~=0)
                 for h=1:a
                     if(label(i,j)~=r_label(1,h))
                         not_before=1;
                     else
                         not_before=0;
                         break
                     end
                 end
                 if not_before==1
                     r_label(1,a)=label(i,j);
                     a=a+1;
                 end
             end
        end 
    end 
end
color(1,:)=2;

== matlab function Audi_A8_1/ENABLED/PPS Model/Radar detection/Straight road segment/Relative velocity2/Embedded MATLAB Function1 ==
  data: r input double; yp2 output double; yp1 input double; K1 input double; K2 output double; TISdet parameter double; TISMaxRange parameter double
function [yp2, K2] = modif(r, yp1, K1, TISdet, TISMaxRange)
%#eml
% Interpolating yp value.

K2 = K1;
yp2 = yp1;

d = 50;

% Adding point
for i = 1 : TISdet
   if r(i) ~= 150
      K2(i,1:d-1) = K2(i,2:d);
      K2(i,d) = yp1(i);
   end
end

% Choosing what to take
for i = 1 : TISdet
    s = 0;
    suma = 0;
    for j = 1 : 50
        if K2(i,j) ~= 0
            suma = suma + K2(i,j);
            s = s + 1;
        end
    end
    yp2(i) = suma/s;
end

% Returning, if object is not detected
for i = 1: TISdet
    if r(i) == TISMaxRange && yp1(i) == 0
        K2(i,:,:) = zeros(d,1);
        yp2(i) = 0;
    end    
end

== matlab function Audi_A8_1/ENABLED/PPS Model/Radar detection/Straight road segment/Relative velocity2/Translation ==
  data: v input double; xpd input double; xp_dot output double; TISdet parameter double
function xp_dot = trans(v, xpd, TISdet)
%#codegen
%Translation of the value

xp_dot = xpd;
for i = 1 : TISdet
    if xpd(i) == v
        xp_dot(i) =0;
    end
end
end

== matlab function Audi_A8_1/ENABLED/PPS Model/Pedestrian detection/Image processing/Embedded MATLAB Function ==
  data: im output double size=[375 500]; image input double
function im = sub_image(image)
%#eml
im=zeros(size(image,1),size(image,2));
for i=1:size(image,1)
    for j=1:size(image,2)
        if (image(i,j)==0)
            im(i,j)=1;
        else
            im(i,j)=0;
        end
    end
end

== matlab function Audi_A8_1/ENABLED/PPS Model/Pedestrian detection/PEDES ==
  data: CentAlarms output double; PosObj_subim input double; Centroid_subim input double; alarms output double size=TISdet; BBox input double; BBox_det output double; TISdet parameter double
function [CentAlarms,alarms,BBox_det]= pedes(PosObj_subim, Centroid_subim,BBox,TISdet)
%#eml
CentAlarms=int32(zeros(2,size(PosObj_subim,2)));
alarms=zeros(size(PosObj_subim,2),1);
BBox_det=int32(zeros(4,size(BBox,2)));
a=1;
for i=1:size(PosObj_subim,2)
    for j=1:size(Centroid_subim,2)
        if (Centroid_subim(1,j)~=0)||(Centroid_subim(2,j)~=0)
            if (abs(Centroid_subim(2,j)-PosObj_subim(2,i))<15)||(abs(Centroid_subim(1,j)-PosObj_subim(1,i))<15)%(PosObj_subim(1,i))>BBox(1,j)&&(PosObj_subim(1,i))<(BBox(1,j)+BBox(3,j))
                alarms(a,1)=1;
                CentAlarms(:,a)=PosObj_subim(:,i);%Centroid_subim(:,j);
                BBox_det(:,a)=BBox(:,i);
            end
        end
    end
    a=a+1;
end

== matlab function Audi_A8_1/ENABLED/PPS Model/Pedestrian detection/PEDES1 ==
  data: Im input double size=[375 500]; Imout output double size=[375 500 3]
function Imout = imag(Im)
%#eml
Imout=128*ones(size(Im,1),size(Im,2),3);
Imout(:,:,1)=Im;

== matlab function Audi_A8_1/ENABLED/PPS Model/Pedestrian detection/PEDES2 ==
  data: Im input double size=[375 500]; Imout output double size=[375 500 3]
function Imout = imag(Im)
%#eml
Imout=128*ones(size(Im,1),size(Im,2),3);
Imout(:,:,1)=Im;

== matlab function Audi_A8_1/ENABLED/PPS Model/Radar detection/Straight road segment/THETA Derivative1/Deriv correction ==
  data: th input double; thp input double; thd input double; th_dot output double; TISdet parameter double
function th_dot = stopping(th, thp, thd, TISdet)
%#codegen
% Stopping if nothing is detected.

th_dot = thd;
for i = 1 : TISdet
    if (th(i)==0 && thp(i)~=0) || (th(i)~=0 && thp(i)==0)
        th_dot(i) = 0;
    end
end
end

== matlab function Audi_A8_1/ENABLED/PPS Model/Radar detection/Straight road segment/THETA Derivative1/Theta extrapolation ==
  data: r input double; th1 input double; th2 output double; thd input double; time input double; K1 input double; K2 output double; TISdet parameter double; TISMaxRange parameter double
function [th2, K2] = modif(r, th1, thd, time, K1, TISdet, TISMaxRange)
%#codegen
% Interpolating theta value.

K2 = K1;
th2 = th1;

d = 10;

% Finding points used in interpolation/extrapolation.
for i = 1 : TISdet
    if thd(i) ~= 0
        K2(i,1:d-1,:) = K2(i,2:d,:);
        K2(i,  d,1) = time;
        K2(i,  d,2) = th1(i);
    end
end

% Extrapolation
for i = 1 : TISdet
    j = 1;
    while j < d+1 && K2(i,j,1) == 0
        j = j + 1;
    end
    
    if j > d-2
        th2(i) = th1(i);
    else
        th2(i) = interp1(K2(i,d-2:d,1),K2(i,d-2:d,2),time,'linear','extrap');
    end
end

% Returning, if object is not detected
for i = 1: TISdet
    if r(i) == TISMaxRange && th1(i) == 0
        K2(i,:,:) = zeros(d,2);
        th2(i) = 0;
    end    
end

end

== matlab function Audi_A8_1/ENABLED/PPS Model/Pedestrian detection/PEDES5 ==
  data: blob_subim_proces output double; sub_im input double size=[375 500]; limx_inf input double; limy_inf input double; im_x input double; im_y input double
function blob_subim_proces = blob_subim(sub_im, limx_inf, limy_inf,im_x,im_y)
%#eml
blob_subim_proces=single(zeros(375,500));

limx_sup=limx_inf+im_x;
limy_sup=limy_inf+im_y;

% Assigned the superior and inferior limit 
limx_sup_sorted=max([limx_sup limx_inf]);
limx_inf_sorted=min([limx_sup limx_inf]);
limy_inf_sorted=min([limy_sup limy_inf]);
limy_sup_sorted=max([limy_sup limy_inf]);


[nn, mm] = size( sub_im );
if ( nn <= 3 ) && ( mm <= 3 )
    sub_im = 0;
    % Create a zeros matrix of size (im_y,im_x)
    if im_x~=0 || im_y~=0
        im_x=abs(im_x);
        im_y=abs(im_y);
        assert(im_x<1000);
        assert(im_y<1000);
        sub_im=zeros(im_y+1,im_x+1);
    end
end


blob_subim_proces(limy_inf_sorted:limy_sup_sorted,limx_inf_sorted:limx_sup_sorted)=sub_im;

== matlab function BMW_Z3_1/ENABLED/PPS Model/Pedestrian detection/Blob Analysis/Embedded MATLAB Function1 ==
  data: centroid input double; centout output double; bbox input double; bboxout output double; majoraxis input double; minoraxis input double; orientation input double; eccentricity input double; label input double; label_out output double size=[400 550]; im_x input double; im_y input double; posObj_subim input double; liminf_x input double; liminf_y input double; posObj_im output double
function [centout,bboxout,label_out,posObj_im] = select_blobs(centroid,bbox,majoraxis,minoraxis,orientation,eccentricity,label,im_x,im_y,posObj_subim, liminf_x,liminf_y)
%#eml
a=1;
centroid=int32(centroid);
centout=int32(zeros(2,size(centroid,2)));
bboxout=int32(zeros(4,size(bbox,2)));
label_out=zeros(size(label,1),size(label,2));
posObj_im=posObj_subim;
for i=1:size(posObj_subim,2)
    posObj_im(:,i)=posObj_subim(:,i)+[liminf_y;liminf_x];
end

for i=1:size(orientation,2)
    touch=0;
    if orientation(1,i)>=180
         or_val=360-orientation(1,i);
     else
         or_val=orientation(1,i);
     end
     lr=bbox(1,i)+1;
     lh=lr+bbox(3,i)-1;
     lc=bbox(2,i)+1;
     lw=lc+bbox(4,i)-1;
      if (bbox(1,i)==0)
          touch=touch+1;
      end
      if (bbox(2,i)==0)
          touch=touch+1;
      end
      if(im_y-centroid(1,i)-(bbox(4,i)/2)<2)
          touch=touch+1;
      end
      if (im_x-centroid(2,i)-(bbox(3,i)/2)<2)
          touch=touch+1;
      end
     
     if (abs(or_val)>55)&&(abs(or_val)<145)&&((majoraxis(i)/minoraxis(i))>1.5)&&((majoraxis(i)/minoraxis(i))<3)&&(eccentricity(i)>0)&&(eccentricity(i)<1)&&(touch<2)
         bboxout(1:2,a)= bbox(1:2,i)+int32([liminf_y;liminf_x]);
         bboxout(3:4,a)= bbox(3:4,i);
         centout(:,a)= centroid(:,i)+int32([liminf_y;liminf_x]);
         label_out(lr:lh,lc:lw)=a;
         a=a+1;
     else
        label_out(lr:lh,lc:lw)=0;
     end
end

== matlab function BMW_Z3_1/ENABLED/PPS Model/Pedestrian detection/Blob Analysis/Embedded MATLAB Function2 ==
  data: nbboxout input double; label input double; r_label output double; color output double
function [r_label,color] = r_labels(nbboxout,label)
%#eml
n=size(nbboxout,2);
r_label=zeros(1,n);
color=zeros(1,n);
not_before=1;
a=1;
for i=1:size(label,1)
    for j=1:size(label,2)
        if (a==1)
            if (label(i,j)~=0)
                r_label(1,a)=label(i,j);
                a=a+1;
            end
        else
             if (label(i,j)~=0)
                 for h=1:a
                     if(label(i,j)~=r_label(1,h))
                         not_before=1;
                     else
                         not_before=0;
                         break
                     end
                 end
                 if not_before==1
                     r_label(1,a)=label(i,j);
                     a=a+1;
                 end
             end
        end 
    end 
end
color(1,:)=2;

== matlab function BMW_Z3_1/ENABLED/PPS Model/Pedestrian detection/Blob Analysis/MATLAB Function ==
  data: u input double; y output double
function y = fcn(u)
%#codegen

y = u(1:2, :);

== matlab function BMW_Z3_1/ENABLED/PPS Model/Pedestrian detection/Blob Analysis/PEDES1 ==
  data: inpoints output double; pts input double
function inpoints= points(pts)
%#eml
inpoints = pts;
inpoints(1, :)=pts(2, :);
inpoints(2, :)=pts(1, :);

for i = 1 : size(inpoints, 2)
    if inpoints(1, i) ~= -1
        inpoints(1, i)=inpoints(1, i) +1;
    end
    if inpoints(2, i) ~= -1
        inpoints(2, i)=inpoints(2, i) +1;
    end
end

== matlab function BMW_Z3_1/ENABLED/PPS Model/Pedestrian detection/Blob Analysis/PEDES2 ==
  data: inpoints output double; pts input double
function inpoints= points(pts)
%#eml
inpoints = pts;
inpoints(1, :)=pts(2, :);
inpoints(2, :)=pts(1, :);
inpoints(3, :)=pts(4, :);
inpoints(4, :)=pts(3, :);

for i = 1 : size(inpoints, 2)
    if inpoints(1, i) ~= -1
        inpoints(1, i)=inpoints(1, i) -1;
    end
    if inpoints(2, i) ~= -1
        inpoints(2, i)=inpoints(2, i) -1;
    end
end

== matlab function BMW_Z3_1/ENABLED/PPS Model/Pedestrian detection/Blob Analysis/PEDES3 ==
  data: inpoints output double; pts input double
function inpoints= points(pts)
%#eml
inpoints = pts;
inpoints(1, :)=pts(2, :);
inpoints(2, :)=pts(1, :);
for i = 1 : size(inpoints, 2)
    if inpoints(1, i) ~= -1
        inpoints(1, i)=inpoints(1, i) -1;
    end
    if inpoints(2, i) ~= -1
        inpoints(2, i)=inpoints(2, i) -1;
    end
end

== matlab function BMW_Z3_1/ENABLED/PPS Model/Pedestrian detection/Blob Analysis/PEDES4 ==
  data: inpoints output double; pts input double
function inpoints= points(pts)
%#eml
inpoints = pts;
inpoints(1, :)=pts(2, :);
inpoints(2, :)=pts(1, :);
inpoints(3, :)=pts(4, :);
inpoints(4, :)=pts(3, :);

for i = 1 : size(inpoints, 2)
    if inpoints(1, i) ~= -1
        inpoints(1, i)=inpoints(1, i) +1;
    end
    if inpoints(2, i) ~= -1
        inpoints(2, i)=inpoints(2, i) +1;
    end
end

== matlab function BMW_Z3_1/ENABLED/PPS Model/Pedestrian detection/Image processing/Embedded MATLAB Function ==
  data: im output double size=[375 500]; image input double
function im = sub_image(image)
%#eml
im=zeros(size(image,1),size(image,2));
for i=1:size(image,1)
    for j=1:size(image,2)
        if (image(i,j)==0)
            im(i,j)=1;
        else
            im(i,j)=0;
        end
    end
end
